simulink model "Serial_Comm"  (R2022a)
settings: Solver=VariableStepAuto  StartTime=0.0  StopTime=10.0  RelTol=1e-3
libraries: instrumentseriallib x2
settings Model: Creator=alake  LastModifiedBy=alake

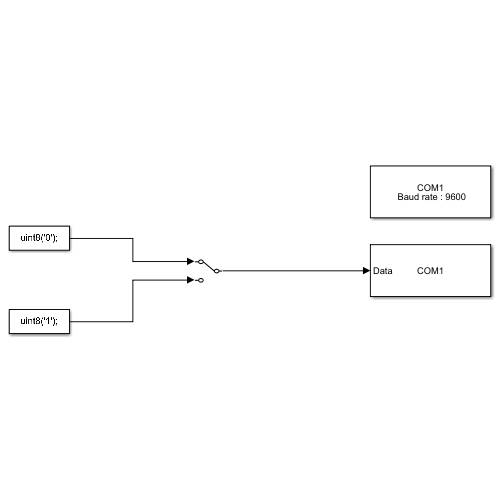
[thumbnail: Simulink's stored preview of the top-level diagram]
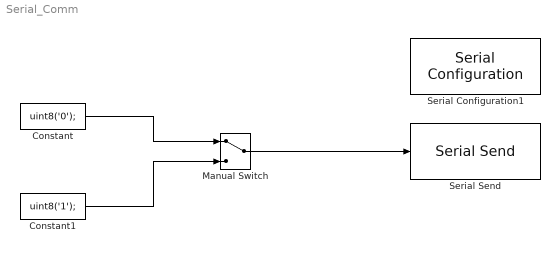
== system Serial_Comm ==
  Constant : Constant  Value=uint8('0');
  Constant1 : Constant  Value=uint8('1');
  Manual Switch : ManualSwitch
  Serial Configuration1 : instrumentseriallib/Serial Configuration  Priority=-200000  PortSel=COM1  Port=COM1  ComPort=COM1  BaudRate=9600  DataBits=8  Parity=none  StopBits=1  ByteOrder=little-endian  FlowControl=none  Timeout=10  SimulateUsing=Interpreted execution  BlockInModel=on  aMode=1
      settings: SourceProductBaseCode=OT,IC,MT
  Serial Send : instrumentseriallib/Serial Send  Priority=1  PortSel=COM1  Port=COM1  ComPort=COM1  Header=[]  Terminator=<none>  CustomTerminator=[]  EnableBlockingMode=on  SimulateUsing=Interpreted execution  BlockInModel=on  aMode=1
      settings: SourceProductBaseCode=OT,IC,MT
  wires:
  Manual Switch/1 -> Serial Send/1
  Constant/1 -> Manual Switch/1
  Constant1/1 -> Manual Switch/2
